simulink model "opFeedback_delta"  (R2018a)
settings: Solver=VariableStepAuto  StartTime=0.0  StopTime=10.0  RelTol=1e-3
undefined symbols (not defined in the file or in its folder): frictionMatrix, Gxmatrix, Mmatrix, Nmatrix
settings Model: Creator=klay  LastModifiedBy=augus
settings CodeAppCC: StateflowObjectComments=on

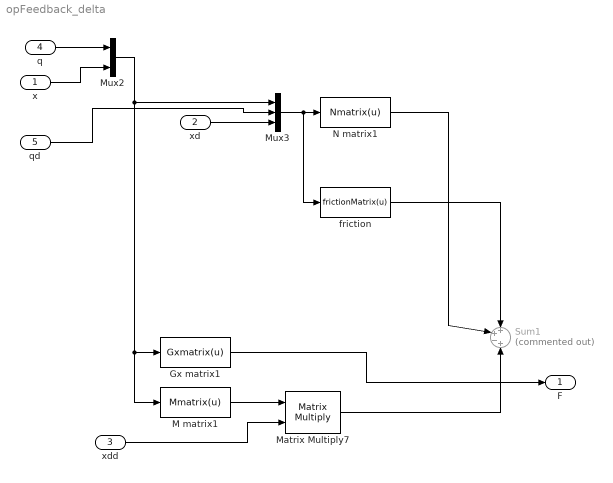
== system opFeedback_delta ==
  x : Inport  PortDimensions=3
  xd : Inport  Port=2  PortDimensions=3
  xdd : Inport  Port=3  PortDimensions=3
  q : Inport  Port=4  PortDimensions=3
  qd : Inport  Port=5  PortDimensions=3
  Gx matrix1 : MATLABFcn  MATLABFcn=Gxmatrix(u)  Output1D=off
  M matrix1 : MATLABFcn  MATLABFcn=Mmatrix(u)  Output1D=off
  Matrix Multiply7 : Product  Multiplication=Matrix(*)
  Mux2 : Mux  Inputs=2
  Mux3 : Mux  Inputs=3
  N matrix1 : MATLABFcn  MATLABFcn=Nmatrix(u)  Output1D=off
  Sum1 : Sum  Commented=on  Inputs=++-+
  friction : MATLABFcn  MATLABFcn=frictionMatrix(u)  Output1D=off
  F : Outport  PortDimensions=3
  wires:
  x/1 -> Mux2/2
  Mux2/1 -> M matrix1/1, Gx matrix1/1, Mux3/1
  xd/1 -> Mux3/3
  M matrix1/1 -> Matrix Multiply7/1
  xdd/1 -> Matrix Multiply7/2
  Mux3/1 -> friction/1, N matrix1/1
  N matrix1/1 -> Sum1/2
  friction/1 -> Sum1/1
  Matrix Multiply7/1 -> Sum1/4
  q/1 -> Mux2/1
  qd/1 -> Mux3/2
  Gx matrix1/1 -> F/1
